simulink model "bh_a_spring_mass_model"  (R2017a)
settings: Solver=ode45  StartTime=0.0  StopTime=10.0  RelTol=1e-7
settings Model: Creator=bhorton  LastModifiedBy=bhorton

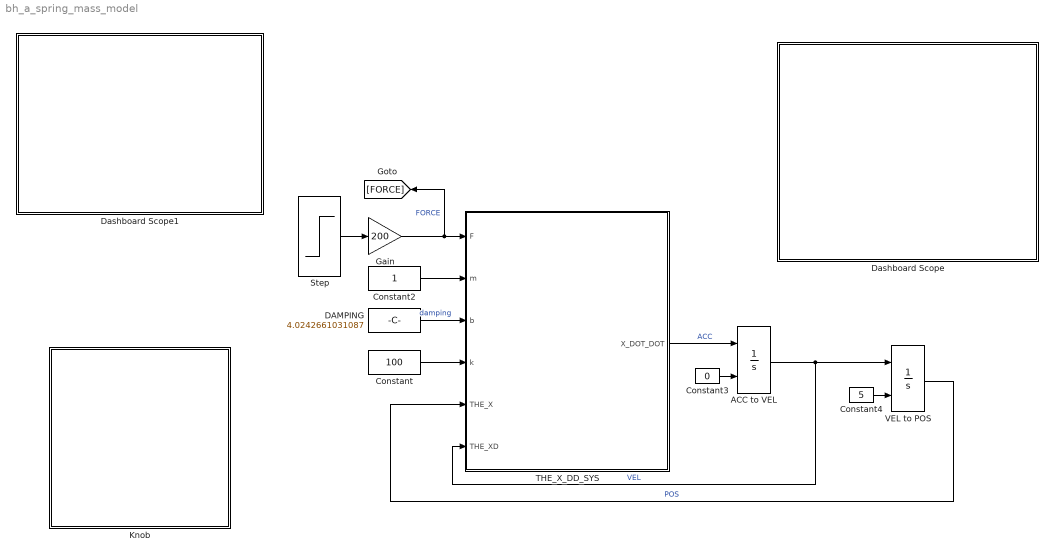
== system bh_a_spring_mass_model ==
  ACC to VEL : Integrator  InitialConditionSource=external
  Constant : Constant  Value=100
  Constant2 : Constant
  Constant3 : Constant  Value=0
  Constant4 : Constant  Value=5
  DAMPING : Constant  Value=4.0242661031087
  Dashboard Scope : Subsystem  DialogController=hmiCreateDDGDialog  IsWebBlock=on  mask(MWDashboardBlock){webBlockId=47d7a76a-e090-4f37-bb13-c45fee118520, webBlockType=sdiscope, ShowInitialText=on, HMISrcModelName=bh_a_spring_mass_model}
      mask prompts: webBlockId "WebBlock Id"; webBlockType "WebBlock Type"; HMISrcModelName "Source Model"
      mask help: SimulinkHMI:dialogs:HMIScopeDialogDesc
      mask Help: helpview([docroot '/mapfiles/simulink.map'], 'hmi_scope')
      mask Display:
      | if strcmp(get_param(bdroot(gcb),'BlockDiagramType'), 'library')
      |     image([(matlabroot) '/toolbox/simulink/hmi/icons/DashboardScope.png']);
      | end
  Dashboard Scope1 : Subsystem  DialogController=hmiCreateDDGDialog  IsWebBlock=on  mask(MWDashboardBlock){webBlockId=8ddedbd7-6b40-4d71-b8ad-862d34055e22, webBlockType=sdiscope, ShowInitialText=on, HMISrcModelName=bh_a_spring_mass_model}
      mask prompts: webBlockId "WebBlock Id"; webBlockType "WebBlock Type"; HMISrcModelName "Source Model"
      mask help: SimulinkHMI:dialogs:HMIScopeDialogDesc
      mask Help: helpview([docroot '/mapfiles/simulink.map'], 'hmi_scope')
      mask Display:
      | if strcmp(get_param(bdroot(gcb),'BlockDiagramType'), 'library')
      |     image([(matlabroot) '/toolbox/simulink/hmi/icons/DashboardScope.png']);
      | end
  Gain : Gain  Gain=200
  Knob : Subsystem  DialogController=hmiCreateDDGDialog  IsWebBlock=on  mask(MWDashboardBlock){webBlockId=7851c9e5-dfa2-459a-b2bd-c1eacf40fcae, webBlockType=continuousknob, ShowInLibBrowser=on, ShowInitialText=on, HMISrcModelName=bh_a_spring_mass_model}
      mask prompts: webBlockId "WebBlock Id"; webBlockType "WebBlock Type"; HMISrcModelName "Source Model"
      mask help: SimulinkHMI:dialogs:ContinuousKnobDialogDesc
      mask Help: helpview([docroot '/mapfiles/simulink.map'], 'hmi_knob')
      mask Display:
      | if strcmp(get_param(bdroot(gcb),'BlockDiagramType'), 'library')
      |     image([(matlabroot) '/toolbox/simulink/hmi/icons/ContinuousKnob.png']);
      | end
  Step : Step  Time=5  SampleTime=0
  THE_X_DD_SYS : MATLAB Function  TreatAsAtomicUnit=on
  VEL to POS : Integrator  InitialConditionSource=external
  wires:
  Step/1 -> Gain/1
  Gain/1 -> THE_X_DD_SYS/1(F), [FORCE]  "FORCE"
  THE_X_DD_SYS/1(X_DOT_DOT) -> ACC to VEL/1  "ACC"
  ACC to VEL/1 -> THE_X_DD_SYS/6(THE_XD), VEL to POS/1  "VEL"
  VEL to POS/1 -> THE_X_DD_SYS/5(THE_X)  "POS"
  Constant2/1 -> THE_X_DD_SYS/2(m)
  DAMPING/1 -> THE_X_DD_SYS/3(b)  "damping"
  Constant/1 -> THE_X_DD_SYS/4(k)
  Constant3/1 -> ACC to VEL/2
  Constant4/1 -> VEL to POS/2

== system bh_a_spring_mass_model/Dashboard Scope ==

== system bh_a_spring_mass_model/Dashboard Scope1 ==

== system bh_a_spring_mass_model/Knob ==

== matlab function bh_a_spring_mass_model/THE_X_DD_SYS ==
  data: F input; X_DOT_DOT output; m input; b input; k input; THE_X input; THE_XD input
function X_DOT_DOT = THE_X_DD_SYS(F,m,b,k,THE_X,THE_XD)
%#codegen

%    This function was generated by the Symbolic Math Toolbox version 7.2.
%    27-Mar-2017 09:20:04

X_DOT_DOT = -(-F+THE_XD.*b+THE_X.*k)./m;
